simulink model "gm_uz_threephase_VSD_transformation"  (R2021b)
settings: Solver=FixedStepAuto  StartTime=0.0  StopTime=inf  RelTol=1e-3
libraries: hdlmdlgenlib x19, dspsigops x5
settings Model: Creator=ts  LastModifiedBy=valen
settings SolverCC: AlgebraicLoopSolver=TrustRegion  AutoInsertRateTranBlk=on
settings DataIOCC: LimitDataPoints=on  SaveOutput=off  SaveTime=off
settings OptimizationCC: BlockReduction=off  ConditionallyExecuteInputs=off  DefaultParameterBehavior=Inlined  InheritOutputTypeSmallerThanSingle=on  LifeSpan=inf
settings DebuggingCC: AlgebraicLoopMsg=error  InheritedTsInSrcMsg=none  SingleTaskRateTransMsg=error  AllowSymbolicDim=off  StrictBusMsg=ErrorOnBusTreatedAsVector  SFUnexpectedBacktrackingDiag=warning  SFNoUnconditionalDefaultTransitionDiag=warning  SFExecutionAtInitializationDiag=none  SFMachineParentedDataDiag=warning  ArithmeticOperatorsInVariantConditions=warning
settings HardwareCC: ProdBitPerPointer=32  ProdBitPerSizeT=32  ProdBitPerPtrDiffT=32  ProdLargestAtomicFloat=None  ProdIntDivRoundTo=Undefined  ProdEndianess=Unspecified  ProdWordSize=32  ProdHWDeviceType=ASIC/FPGA->ASIC/FPGA  ProdEqTarget=off
settings SFSimCC: SimUseLocalCustomCode=off  CustomCodeUndefinedFunction=UseInterfaceOnly
settings RTWCC: RTWUseLocalCustomCode=off
settings CodeAppCC: StateflowObjectComments=on
settings GRTTargetCC: TargetLangStandard=C89/C90 (ANSI)
settings ConfigComp: CovScope=ReferencedModels  CovMetricSettings=dw  CovSaveCumulativeToWorkspaceVar=on  CovSaveSingleToWorkspaceVar=on  CovExternalEMLEnable=off  CovSFcnEnable=off

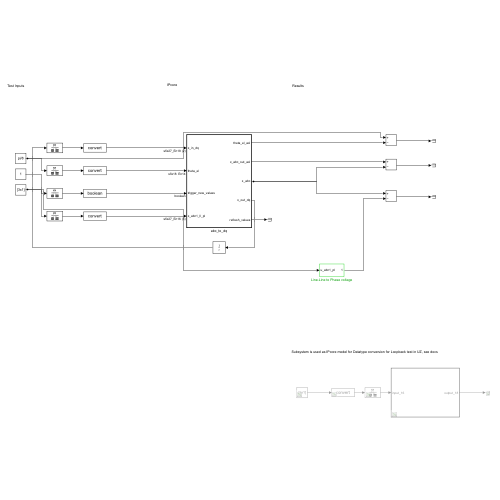
[thumbnail: Simulink's stored preview of the top-level diagram]
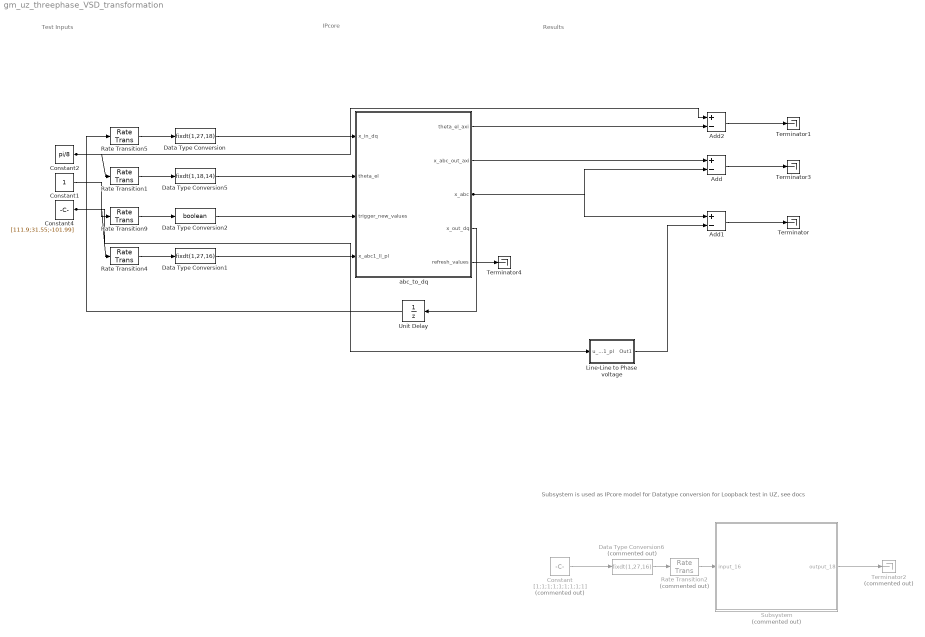
== system gm_uz_threephase_VSD_transformation ==
  note: IPcore
  note: Test Inputs
  note: Results
  note: Subsystem is used as IPcore model for Datatype conversion for Loopback test in UZ, see docs
  Add : Sum  Inputs=+-
  Add1 : Sum  Inputs=+-
  Add2 : Sum  Inputs=+-
  Constant : Constant  Commented=on  Value=[1;1;1;1;1;1;1;1;1]
  Constant1 : Constant
  Constant2 : Constant  Value=pi/8
  Constant4 : Constant  Value=[111.9;31.55;-101.99]
  Data Type Conversion : DataTypeConversion  OutDataTypeStr=fixdt(1,27,18)
  Data Type Conversion1 : DataTypeConversion  OutDataTypeStr=fixdt(1,27,16)
  Data Type Conversion2 : DataTypeConversion  OutDataTypeStr=boolean
  Data Type Conversion5 : DataTypeConversion  OutDataTypeStr=fixdt(1,18,14)
  Data Type Conversion6 : DataTypeConversion  Commented=on  OutDataTypeStr=fixdt(1,27,16)
  Line-Line to Phase voltage : Subsystem
  Rate Transition{1,4..5,9} (4 alike) : RateTransition  OutPortSampleTime=ts_uz_ninephase_VSD_transformation
  Rate Transition2 : RateTransition  Commented=on  OutPortSampleTime=ts_uz_ninephase_VSD_transformation
  Subsystem : Subsystem  Commented=on  TreatAsAtomicUnit=on
  Terminator{,1,3..4} (4 alike) : Terminator
  Terminator2 : Terminator  Commented=on
  Unit Delay : UnitDelay  SampleTime=-1  HasFrameUpgradeWarning=on
  abc_to_dq : Subsystem  TreatAsAtomicUnit=on
  wires:
  abc_to_dq/5(refresh_values) -> Terminator4/1
  Rate Transition2/1 -> Subsystem/1(input_16)
  Data Type Conversion6/1 -> Rate Transition2/1
  Constant/1 -> Data Type Conversion6/1
  Subsystem/1(output_18) -> Terminator2/1
  Line-Line to Phase voltage/1(Out1) -> Add1/2
  Unit Delay/1 -> Rate Transition5/1
  Add/1 -> Terminator3/1
  Constant4/1 -> Rate Transition4/1, Line-Line to Phase voltage/1(u_abc1_pl)
  Add2/1 -> Terminator1/1
  abc_to_dq/1(theta_el_axi) -> Add2/2
  Add1/1 -> Terminator/1
  abc_to_dq/2(x_abc_out_axi) -> Add/1
  abc_to_dq/3(x_abc) -> Add/2, Add1/1
  Constant2/1 -> Rate Transition1/1, Add2/1
  abc_to_dq/4(x_out_dq) -> Unit Delay/1
  Rate Transition1/1 -> Data Type Conversion5/1
  Data Type Conversion5/1 -> abc_to_dq/2(theta_el)
  Constant1/1 -> Rate Transition9/1
  Rate Transition9/1 -> Data Type Conversion2/1
  Data Type Conversion2/1 -> abc_to_dq/3(trigger_new_values)
  Rate Transition4/1 -> Data Type Conversion1/1
  Rate Transition5/1 -> Data Type Conversion/1
  Data Type Conversion1/1 -> abc_to_dq/4(x_abc1_ll_pl)
  Data Type Conversion/1 -> abc_to_dq/1(x_in_dq)

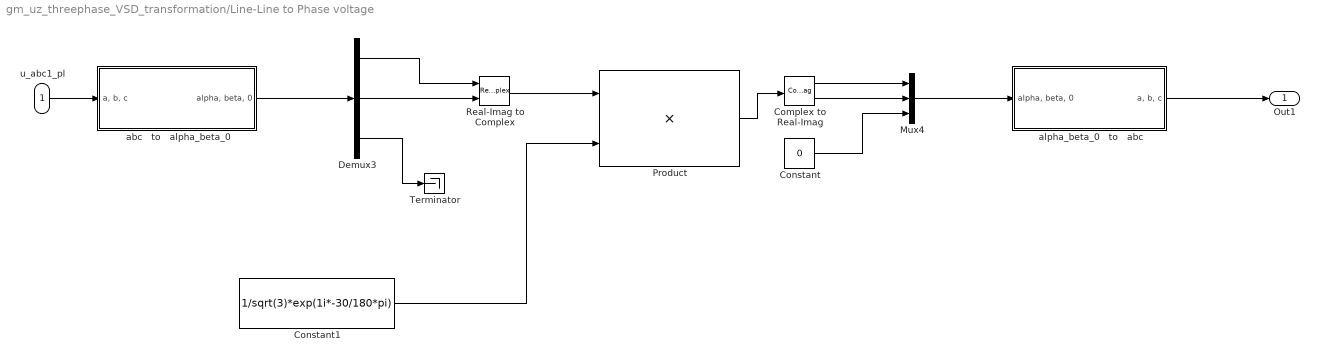
== system gm_uz_threephase_VSD_transformation/Line-Line to Phase voltage ==
  u_abc1_pl : Inport
  Complex to Real-Imag : ComplexToRealImag
  Constant : Constant  Value=0  OutDataTypeStr=fixdt(1,27,16)  SampleTime=-1
  Constant1 : Constant  Value=1/sqrt(3)*exp(1i*-30/180*pi)  OutDataTypeStr=fixdt(1,18,16)  SampleTime=-1
  Demux3 : Demux  Outputs=3
  Mux4 : Mux  Inputs=3
  Product : Product  OutDataTypeStr=fixdt(1,27,16)
  Real-Imag to Complex : RealImagToComplex
  Terminator : Terminator
  abc   to   alpha_beta_0 : Subsystem
  alpha_beta_0   to   abc : Subsystem
  Out1 : Outport
  wires:
  Constant1/1 -> Product/2
  alpha_beta_0   to   abc/1("a, b, c") -> Out1/1
  abc   to   alpha_beta_0/1("alpha, beta, 0 ") -> Demux3/1
  Demux3/3 -> Terminator/1
  u_abc1_pl/1 -> abc   to   alpha_beta_0/1("a, b, c")
  Constant/1 -> Mux4/3
  Complex to Real-Imag/2 -> Mux4/2
  Demux3/1 -> Real-Imag to Complex/1
  Real-Imag to Complex/1 -> Product/1
  Product/1 -> Complex to Real-Imag/1
  Mux4/1 -> alpha_beta_0   to   abc/1("alpha, beta, 0  ")
  Complex to Real-Imag/1 -> Mux4/1
  Demux3/2 -> Real-Imag to Complex/2

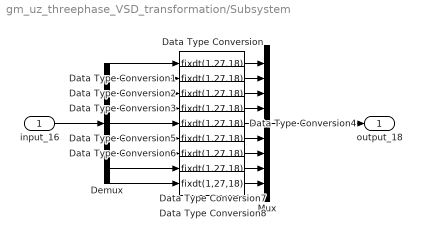
== system gm_uz_threephase_VSD_transformation/Subsystem ==
  input_16 : Inport
  Data Type Conversion{,1..8} (9 alike) : DataTypeConversion  OutDataTypeStr=fixdt(1,27,18)
  Demux : Demux  Outputs=9
  Mux : Mux  Inputs=9
  output_18 : Outport
  wires:
  Mux/1 -> output_18/1
  Data Type Conversion8/1 -> Mux/9
  Data Type Conversion7/1 -> Mux/8
  Data Type Conversion6/1 -> Mux/7
  Data Type Conversion5/1 -> Mux/6
  Data Type Conversion4/1 -> Mux/5
  Data Type Conversion3/1 -> Mux/4
  Data Type Conversion2/1 -> Mux/3
  Data Type Conversion1/1 -> Mux/2
  Data Type Conversion/1 -> Mux/1
  Demux/9 -> Data Type Conversion8/1
  Demux/8 -> Data Type Conversion7/1
  Demux/7 -> Data Type Conversion6/1
  Demux/4 -> Data Type Conversion3/1
  Demux/5 -> Data Type Conversion4/1
  Demux/6 -> Data Type Conversion5/1
  Demux/3 -> Data Type Conversion2/1
  Demux/2 -> Data Type Conversion1/1
  Demux/1 -> Data Type Conversion/1
  input_16/1 -> Demux/1

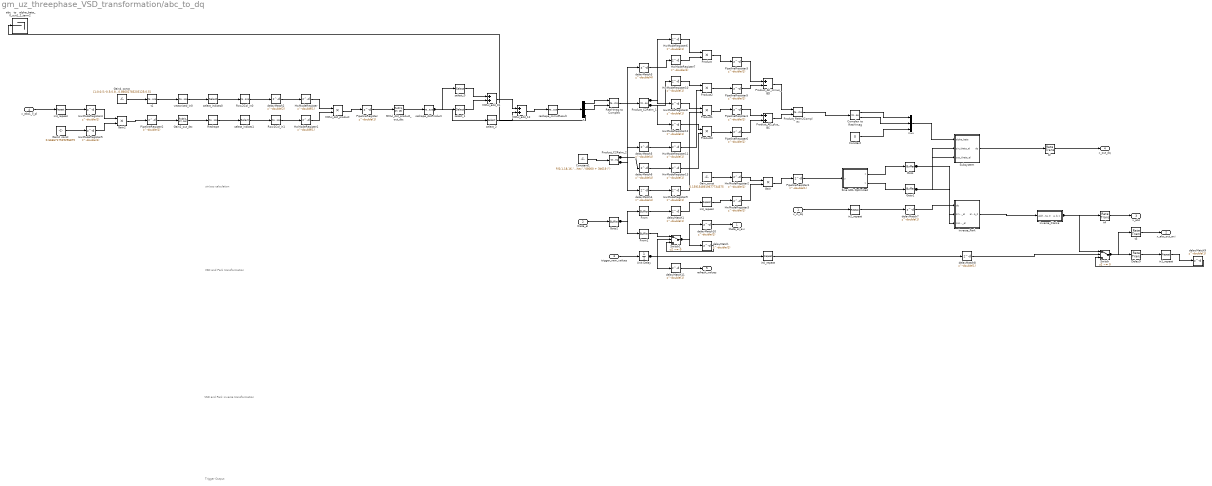
== system gm_uz_threephase_VSD_transformation/abc_to_dq ==
  note: sin/cos calculation
  note: VSD and Park transformation
  note: VSD and Park inverse transformation
  note: Trigger Output
  x_in_dq : Inport  OutDataTypeStr=fixdt(1, 27, 18)  PortDimensions=[2]  SampleTime=1e-06
  theta_el : Inport  Port=2  OutDataTypeStr=fixdt(1, 18, 14)  PortDimensions=1  SampleTime=1e-06
  trigger_new_values : Inport  Port=3  OutDataTypeStr=boolean  PortDimensions=1  SampleTime=1e-06
  x_abc1_ll_pl : Inport  Port=4  OutDataTypeStr=fixdt(1, 27, 16)  PortDimensions=[3]  SampleTime=1e-06
  Complex to Real-Imag : ComplexToRealImag  SampleTime=1e-08
  Constant : Constant  Value=0  OutDataTypeStr=fixdt(1, 27, 16)  SampleTime=1e-08
  Constant1 : Constant  Value="fi(0,1,18,16,\"hex\",\"08000 + 3b619 i\")"  OutDataTypeStr=fixdt(1, 18, 16)  SampleTime=1e-08
  Delay9 : RateTransition  OutPortSampleTimeOpt=Multiple of input port sample time  OutPortSampleTimeMultiple=100
  From : hdlmdlgenlib/Buffer
      settings: SourceProductBaseCode=SL
  From1 : hdlmdlgenlib/Buffer
      settings: SourceProductBaseCode=SL
  Gain : Product  Inputs=**  OutDataTypeStr=fixdt(1, 18, 16)  SampleTime=1e-08
  Gain2 : Product  Inputs=**  OutDataTypeStr=fixdt(1, 45, 32)  SampleTime=1e-08
  Gain2_const : Constant  Value=0.6666717529296875  OutDataTypeStr=fixdt(1, 18, 16)  SampleTime=1e-08
  Gain2_out_dtc : DataTypeConversion  OutDataTypeStr=fixdt(1, 27, 16)  SampleTime=1e-08  SaturateOnIntegerOverflow=on
  Gain4_const : Constant  Value=[1;0;0.5;-0.5;0.86602783203125;0.5;-0.5;-0.86602783203125;0.5]  OutDataTypeStr=fixdt(1, 18, 16)  SampleTime=1e-08
  Gain_const : Constant  Value=0.1591548919677734375  OutDataTypeStr=fixdt(1, 18, 19)  SampleTime=1e-08
  Goto : hdlmdlgenlib/Buffer
      settings: SourceProductBaseCode=SL
  Goto1 : hdlmdlgenlib/Buffer
      settings: SourceProductBaseCode=SL
  Goto2 : hdlmdlgenlib/Buffer
      settings: SourceProductBaseCode=SL
  HwModeRegister{,1..13} (14 alike) : Delay  DelayLength=double(1)  InitialCondition=0  SampleTime=1e-08
  MMul_add_01 : Sum  OutDataTypeStr=fixdt(1, 27, 16)  SaturateOnIntegerOverflow=on  SampleTime=1e-08
  MMul_add_12 : Sum  OutDataTypeStr=fixdt(1, 27, 16)  SaturateOnIntegerOverflow=on  SampleTime=1e-08
  MMul_dot_product : Product  Inputs=**  OutDataTypeStr=fixdt(1, 45, 32)  SampleTime=1e-08
  MMul_dot_product_out_dtc : DataTypeConversion  OutDataTypeStr=fixdt(1, 27, 16)  SampleTime=1e-08  SaturateOnIntegerOverflow=on
  PipelineRegister{,1..6} (7 alike) : Delay  DelayLength=double(1)  InitialCondition=0  SampleTime=1e-08
  Product{,1..3} (4 alike) : Product  Inputs=**  OutDataTypeStr=fixdt(1, 27, 16)  SampleTime=1e-08
  Product_AC_minus_BD : Sum  Inputs=+-  OutDataTypeStr=fixdt(1, 27, 16)  SampleTime=1e-08
  Product_AD_plus_BC : Sum  OutDataTypeStr=fixdt(1, 27, 16)  SampleTime=1e-08
  Product_C2ReIm_1 : ComplexToRealImag  SampleTime=1e-08
  Product_C2ReIm_2 : ComplexToRealImag  SampleTime=1e-08
  Product_ReIm2Complex : RealImagToComplex  SampleTime=1e-08
  Real-Imag to Complex : RealImagToComplex  ConstantPart="fi(0,1,27,16,\"hex\",\"0000000\")"  SampleTime=1e-08
  Reshape : Reshape  OutputDimensionality=Column vector (2-D)
  Row2Col_in0 : Reshape  OutputDimensionality=Column vector (2-D)
  Row2Col_in1 : Reshape  OutputDimensionality=Column vector (2-D)
  Sine HDL Optimized : Subsystem  mask(Sine and Cosine HDL optimized block){OutputFormula=sin(2*pi*u) and cos(2*pi*u), NumDataPoints=double(256), TableDataTypeStr=fixdt(0,17,16), SimulateLUTROMDelay=off}
      mask prompts: OutputFormula "Simulink:masks:OutputFormula_MP"; NumDataPoints "HDLShared:hdlshared:CosineHDL_Npts"; TableDataTypeStr "Simulink:blkprm_prompts:TABLE_UNIFIEDDATATYPE"; SimulateLUTROMDelay "HDLShared:hdlshared:CosineHDL_SimulateLUTDelay"
      mask help: Sine and Cosine HDL optimized block using quarter wave symmetry, and HDL friendly settings.
      mask Help: helpview([docroot '/hdlcoder/helptargets.map'],'SineAndCosineHDL_Optimized');
      mask TypeOptions OutputFormula: sin(2*pi*u) | cos(2*pi*u) | exp(j*2*pi*u) | sin(2*pi*u) and cos(2*pi*u)
      mask Display:
      | port_label('input',1,'u')
      | port_label('output',1,'sin(2*pi*u)')
      | port_label('output',2,'cos(2*pi*u)')
      | xpos = 0.35;
      | yoffset = 0.5;
      | if ( SimulateLUTROMDelay )
      |   text(xpos,yoffset,'HDL (Z^{-1})','texmode','on')
      | else
      |    text(xpos,yoffset,'HDL')
      | end
  Subsystem : Subsystem
  Switch : Switch  Criteria=u2 ~= 0  Threshold=double(0)  OutDataTypeStr=fixdt(1, 27, 18)  SampleTime=1e-08
  Switch1 : Switch  Criteria=u2 ~= 0  Threshold=double(0)  OutDataTypeStr=fixdt(1, 18, 14)  SampleTime=1e-06
  Unit Delay : UnitDelay  SampleTime=1e-06
  abc   to   alpha_beta_0_out1_2_term2 : Terminator
  delayMatch{,1,10..11} (4 alike) : Delay  DelayLength=double(1)  InitialCondition=0  SampleTime=1e-06
  delayMatch2 : Delay  DelayLength=double(2)  InitialCondition=0  SampleTime=1e-08
  delayMatch{3..6} (4 alike) : Delay  DelayLength=double(4)  InitialCondition=0  SampleTime=1e-08
  delayMatch7 : Delay  DelayLength=double(1)  InitialCondition=0  SampleTime=1e-08
  delayMatch8 : Delay  DelayLength=double(1)  InitialCondition=0  SampleTime=1e-08
  delayMatch9 : Delay  DelayLength=double(1)  InitialCondition=0  SampleTime=1e-08
  in0_repeat : dspsigops/Repeat  N=double(100)  RateOptions=Allow multirate processing  ic=0  mode=Unused parameter value
  in1_repeat : dspsigops/Repeat  N=double(100)  RateOptions=Allow multirate processing  ic=0  mode=Unused parameter value
  in2_repeat : dspsigops/Repeat  N=double(100)  RateOptions=Allow multirate processing  ic=0  mode=Unused parameter value
  in3_repeat : dspsigops/Repeat  N=double(100)  RateOptions=Allow multirate processing  ic=0  mode=Unused parameter value
  in4_repeat : dspsigops/Repeat  N=double(100)  RateOptions=Allow multirate processing  ic=0  mode=Unused parameter value
  inverse_Clarke : Subsystem
  inverse_Park : Subsystem
  mux : Mux  Inputs=3
  reshape_dotProduct : Reshape  OutputDimensionality=Customize  OutputDimensions=[3,3]
  reshape_mmulResult : Reshape  OutputDimensionality=Customize  OutputDimensions=[3,1]
  select_0 : Selector  NumberOfDimensions=2  SampleTime=1e-08  IndexOptions=Index vector (dialog),Select all  Indices=double(1),[]  OutputSizes=1
  select_1 : Selector  NumberOfDimensions=2  SampleTime=1e-08  IndexOptions=Index vector (dialog),Select all  Indices=double(2),[]  OutputSizes=1
  select_2 : Selector  NumberOfDimensions=2  SampleTime=1e-08  IndexOptions=Index vector (dialog),Select all  Indices=double(3),[]  OutputSizes=1
  select_indices0 : Selector  SampleTime=1e-08  IndexOptions=Index vector (dialog)  Indices=double([1 4 7 2 5 8 3 6 9])  OutputSizes=1
  select_indices1 : Selector  SampleTime=1e-08  IndexOptions=Index vector (dialog)  Indices=double([1 2 3 1 2 3 1 2 3])  OutputSizes=1
  t : Demux  Outputs=3
  t1 : Reshape  OutputDimensionality=Customize  OutputDimensions=[3,3]
  t2 : RateTransition  OutPortSampleTimeOpt=Multiple of input port sample time  OutPortSampleTimeMultiple=100
  t3 : RateTransition  OutPortSampleTimeOpt=Multiple of input port sample time  OutPortSampleTimeMultiple=100
  t4 : RateTransition  OutPortSampleTimeOpt=Multiple of input port sample time  OutPortSampleTimeMultiple=100
  vectorized_in0 : Reshape  OutputDimensionality=Row vector (2-D)
  theta_el_axi : Outport  SampleTime=1e-06
  x_abc_out_axi : Outport  Port=2  SampleTime=1e-06
  x_abc : Outport  Port=3  SampleTime=1e-06
  x_out_dq : Outport  Port=4  SampleTime=1e-06
  refresh_values : Outport  Port=5  SampleTime=1e-06
  wires:
  x_in_dq/1 -> in2_repeat/1
  theta_el/1 -> Goto2/1
  trigger_new_values/1 -> Unit Delay/1
  x_abc1_ll_pl/1 -> in4_repeat/1
  delayMatch1/1 -> in3_repeat/1
  delayMatch11/1 -> refresh_values/1
  delayMatch10/1 -> theta_el_axi/1
  t2/1 -> x_out_dq/1
  t3/1 -> x_abc_out_axi/1
  t4/1 -> x_abc/1
  Switch1/1 -> delayMatch10/1, delayMatch/1
  Unit Delay/1 -> delayMatch11/1, Switch1/2, in0_repeat/1
  delayMatch/1 -> Switch1/3
  Delay9/1 -> in1_repeat/1
  Goto2/1 -> From1/1, From/1
  From1/1 -> Switch1/1
  From/1 -> delayMatch1/1
  Subsystem/1(dq) -> t2/1
  Switch/1 -> t3/1, Delay9/1
  inverse_Clarke/1("a, b, c") -> t4/1, Switch/1
  in0_repeat/1 -> delayMatch8/1
  in1_repeat/1 -> delayMatch9/1
  in2_repeat/1 -> delayMatch7/1
  in3_repeat/1 -> HwModeRegister3/1
  in4_repeat/1 -> HwModeRegister4/1
  PipelineRegister1/1 -> Sine HDL Optimized/1(u)
  Sine HDL Optimized/1(x) -> Goto/1
  Sine HDL Optimized/2(y) -> Goto1/1
  inverse_Park/1(alpha_beta_0) -> inverse_Clarke/1("alpha, beta, 0  ")
  Constant/1 -> mux/3
  mux/1 -> Subsystem/1(alpha_beta)
  Gain2_out_dtc/1 -> Reshape/1
  Reshape/1 -> select_indices1/1
  reshape_mmulResult/1 -> t/1
  Real-Imag to Complex/1 -> Product_C2ReIm_1/1
  Constant1/1 -> Product_C2ReIm_2/1
  Product_ReIm2Complex/1 -> Complex to Real-Imag/1
  Complex to Real-Imag/1 -> mux/1
  Complex to Real-Imag/2 -> mux/2
  delayMatch8/1 -> Switch/2
  delayMatch9/1 -> Switch/3
  delayMatch7/1 -> inverse_Park/1(dq)
  t/1 -> Real-Imag to Complex/1
  t/2 -> Real-Imag to Complex/2
  t/3 -> abc   to   alpha_beta_0_out1_2_term2/1
  t1/1 -> vectorized_in0/1
  vectorized_in0/1 -> select_indices0/1
  select_indices0/1 -> Row2Col_in0/1
  select_indices1/1 -> Row2Col_in1/1
  delayMatch2/1 -> HwModeRegister/1
  Row2Col_in1/1 -> HwModeRegister1/1
  MMul_dot_product_out_dtc/1 -> reshape_dotProduct/1
  reshape_dotProduct/1 -> select_2/1, select_1/1, select_0/1
  select_0/1 -> MMul_add_01/1
  select_1/1 -> MMul_add_01/2
  MMul_add_01/1 -> MMul_add_12/1
  select_2/1 -> MMul_add_12/2
  MMul_add_12/1 -> reshape_mmulResult/1
  Gain4_const/1 -> t1/1
  Gain_const/1 -> HwModeRegister2/1
  Gain2_const/1 -> HwModeRegister5/1
  Product_C2ReIm_1/1 -> HwModeRegister6/1, HwModeRegister8/1
  Product_C2ReIm_1/2 -> HwModeRegister10/1, HwModeRegister12/1
  delayMatch3/1 -> HwModeRegister7/1
  delayMatch4/1 -> HwModeRegister9/1
  PipelineRegister3/1 -> Product_AC_minus_BD/1
  PipelineRegister4/1 -> Product_AD_plus_BC/1
  PipelineRegister5/1 -> Product_AC_minus_BD/2
  PipelineRegister6/1 -> Product_AD_plus_BC/2
  Product_AC_minus_BD/1 -> Product_ReIm2Complex/1
  Product_AD_plus_BC/1 -> Product_ReIm2Complex/2
  PipelineRegister/1 -> MMul_dot_product_out_dtc/1
  PipelineRegister2/1 -> Gain2_out_dtc/1
  Row2Col_in0/1 -> delayMatch2/1
  delayMatch6/1 -> HwModeRegister13/1
  delayMatch5/1 -> HwModeRegister11/1
  Product_C2ReIm_2/2 -> delayMatch5/1, delayMatch4/1
  Product_C2ReIm_2/1 -> delayMatch6/1, delayMatch3/1
  Goto/1 -> inverse_Park/2(sin_theta_el), Subsystem/2(sin_theta_el)
  Goto1/1 -> inverse_Park/3(cos_theta_el), Subsystem/3(cos_theta_el)
  MMul_dot_product/1 -> PipelineRegister/1
  HwModeRegister/1 -> MMul_dot_product/1
  HwModeRegister1/1 -> MMul_dot_product/2
  Gain/1 -> PipelineRegister1/1
  HwModeRegister2/1 -> Gain/1
  HwModeRegister3/1 -> Gain/2
  Gain2/1 -> PipelineRegister2/1
  HwModeRegister4/1 -> Gain2/1
  HwModeRegister5/1 -> Gain2/2
  Product/1 -> PipelineRegister3/1
  HwModeRegister6/1 -> Product/1
  HwModeRegister7/1 -> Product/2
  Product1/1 -> PipelineRegister4/1
  HwModeRegister8/1 -> Product1/1
  HwModeRegister9/1 -> Product1/2
  Product2/1 -> PipelineRegister5/1
  HwModeRegister10/1 -> Product2/1
  HwModeRegister11/1 -> Product2/2
  Product3/1 -> PipelineRegister6/1
  HwModeRegister12/1 -> Product3/1
  HwModeRegister13/1 -> Product3/2

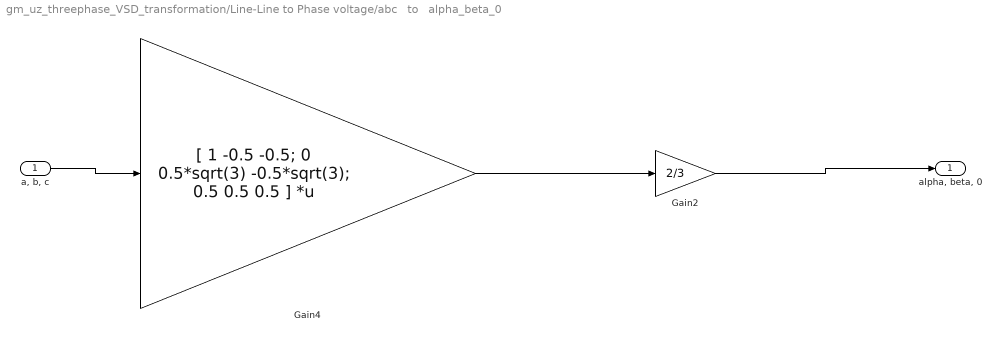
== system gm_uz_threephase_VSD_transformation/Line-Line to Phase voltage/abc   to   alpha_beta_0 ==
  "a, b, c" : Inport  PortDimensions=3
  Gain2 : Gain  Gain=2/3  ParamDataTypeStr=fixdt(1,18,16)  SaturateOnIntegerOverflow=on  OutDataTypeStr=Inherit: Same as input
  Gain4 : Gain  Gain="[ 1   -0.5   -0.5; 0   0.5*sqrt(3)   -0.5*sqrt(3); 0.5  0.5  0.5 ]"  Multiplication=Matrix(K*u) (u vector)  ParamDataTypeStr=fixdt(1,18,16)  OutDataTypeStr=fixdt(1,27,16)  SaturateOnIntegerOverflow=on
  "alpha, beta, 0 " : Outport
  wires:
  Gain4/1 -> Gain2/1
  "a, b, c"/1 -> Gain4/1
  Gain2/1 -> "alpha, beta, 0 "/1

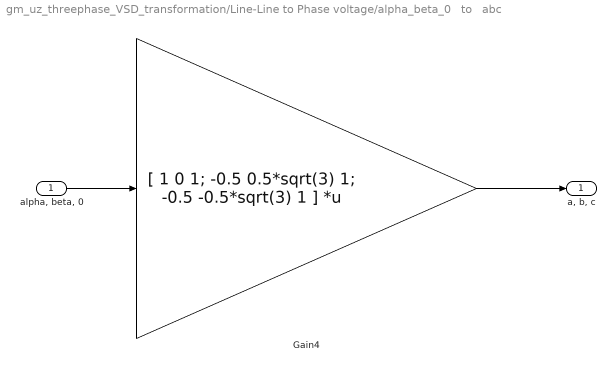
== system gm_uz_threephase_VSD_transformation/Line-Line to Phase voltage/alpha_beta_0   to   abc ==
  "alpha, beta, 0  " : Inport  PortDimensions=3
  Gain4 : Gain  Gain="[ 1 0 1; -0.5   0.5*sqrt(3)  1; -0.5 -0.5*sqrt(3) 1 ]"  Multiplication=Matrix(K*u) (u vector)  ParamDataTypeStr=fixdt(1,18,16)  SaturateOnIntegerOverflow=on  OutDataTypeStr=Inherit: Same as input
  "a, b, c" : Outport
  wires:
  "alpha, beta, 0  "/1 -> Gain4/1
  Gain4/1 -> "a, b, c"/1

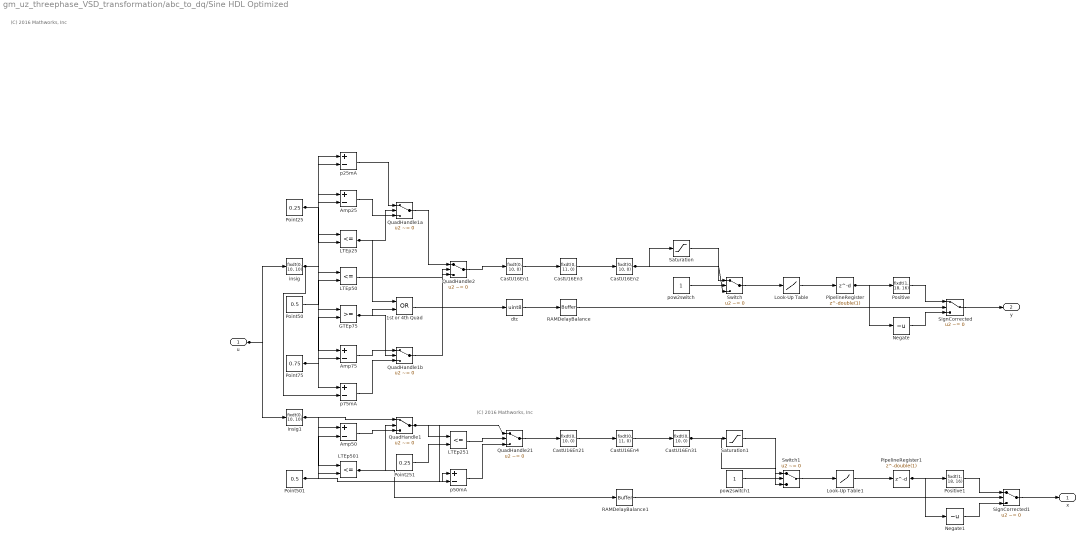
== system gm_uz_threephase_VSD_transformation/abc_to_dq/Sine HDL Optimized ==
  note: (C) 2016 Mathworks, Inc
  note: (C) 2016 Mathworks, Inc
  u : Inport  OutDataTypeStr=fixdt(1, 18, 16)  SampleTime=1e-08
  1st or 4th Quad : Logic  Operator=OR  AllPortsSameDT=off  OutDataTypeStr=boolean  SampleTime=1e-08
  Amp25 : Sum  Inputs=+-  AccumDataTypeStr=fixdt(1, 19, 18)  OutDataTypeStr=fixdt(1, 19, 18)  SampleTime=1e-08
  Amp50 : Sum  Inputs=+-  AccumDataTypeStr=fixdt(1, 19, 18)  OutDataTypeStr=fixdt(1, 19, 18)  SampleTime=1e-08
  Amp75 : Sum  Inputs=+-  AccumDataTypeStr=fixdt(1, 19, 18)  OutDataTypeStr=fixdt(1, 19, 18)  SampleTime=1e-08
  CastU16En1 : DataTypeConversion  OutDataTypeStr=fixdt(0, 10, 0)  ConvertRealWorld=Stored Integer (SI)  SampleTime=1e-08
  CastU16En2 : DataTypeConversion  OutDataTypeStr=fixdt(0, 10, 0)  ConvertRealWorld=Stored Integer (SI)  SampleTime=1e-08  SaturateOnIntegerOverflow=on
  CastU16En21 : DataTypeConversion  OutDataTypeStr=fixdt(0, 10, 0)  ConvertRealWorld=Stored Integer (SI)  SampleTime=1e-08
  CastU16En3 : DataTypeConversion  OutDataTypeStr=fixdt(0, 11, 0)  SampleTime=1e-08
  CastU16En31 : DataTypeConversion  OutDataTypeStr=fixdt(0, 10, 0)  ConvertRealWorld=Stored Integer (SI)  SampleTime=1e-08  SaturateOnIntegerOverflow=on
  CastU16En4 : DataTypeConversion  OutDataTypeStr=fixdt(0, 11, 0)  SampleTime=1e-08
  GTEp75 : RelationalOperator  OutDataTypeStr=boolean  SampleTime=1e-08  RndMeth=Nearest
  LTEp{25,50,251,501} (4 alike) : RelationalOperator  Operator=<=  OutDataTypeStr=boolean  SampleTime=1e-08  RndMeth=Nearest
  Look-Up Table : Lookup_n-D  NumberOfTableDimensions=1  BreakpointsForDimension1="fi(\"numerictype\",numerictype(0,10,0),\"fimath\",fimath(\"RoundingMethod\", \"Floor\",\"OverflowAction\", \"Wrap\",\"ProductMode\",\"FullPrecision\",\"SumMode\",\"FullPrecision\"),\"Value\",\"[0 1 2 3 4 5 6 7 8 9 10 11 12 13 14 15 16 17 18 19 20 21 22 23 24 25 26 27 28 29 30 31 32 33 34 35 36 37 38 39 40 41 42 43 44 45 46 47 48 49 50 51 52 53 54 55 56 57 58 59 60 61 62 63 64 65 66 67 68 69 70 71 72 73 74 75 76 77 78 79 80 81 82 83 84 85 86 87 88 89 90 91 92 93 94 95 96 97 98 99 100 101 102 103 104 105 106 107 108 109 110 111 112 113 114 115 116 117 118 119 120 121 122 123 124 125 126 127 128 129 130 131 132 133 134 135 136 137 138 139 140 141 142 143 144 145 146 147 148 149 150 151 152 153 154 155 156 157 158 159 160 161 162 163 164 165 166 167 168 169 170 171 172 173 174 175 176 177 178 179 180 181 182 183 184 185 186 187 188 189 190 191 192 193 194 195 196 197 198 199 200 201 202 203 204 205 206 207 208 209 210 211 212 213 214 215 216 217 218 219 220 221 222 223 224 225 226 227 228 229 230 231 232 233 234 235 236 237 238 239 240 241 242 243 244 245 246 247 248 249 250 251 252 253 254 255]\")"  Table="reshape(fi(\"numerictype\",numerictype(1,18,16),\"fimath\",fimath(\"RoundingMethod\", \"Floor\",\"OverflowAction\", \"Wrap\",\"ProductMode\",\"FullPrecision\",\"SumMode\",\"FullPrecision\"),\"Value\",\"[0;0.006134033203125;0.01226806640625;0.018402099609375;0.0245361328125;0.030670166015625;0.03680419921875;0.042938232421875;0.049072265625;0.0551910400390625;0.0613250732421875;0.06744384765625;0.0735626220703125;0.079681396484375;0.0858001708984375;0.0919036865234375;0.0980224609375;0.1041259765625;0.1102294921875;0.1163177490234375;0.122406005859375;0.1284942626953125;0.13458251953125;0.140655517578125;0.146728515625;0.152801513671875;0.1588592529296875;0.1649169921875;0.17095947265625;0.177001953125;0.18304443359375;0.1890716552734375;0.1950836181640625;0.20111083984375;0.2071075439453125;0.213104248046875;0.2191009521484375;0.2250823974609375;0.2310638427734375;0.237030029296875;0.24298095703125;0.248931884765625;0.2548675537109375;0.2607879638671875;0.2667083740234375;0.2726287841796875;0.2785186767578125;0.2844085693359375;0.290283203125;0.2961578369140625;0.302001953125;0.3078460693359375;0.3136749267578125;0.3195037841796875;0.3253173828125;0.3311004638671875;0.336883544921875;0.3426666259765625;0.348419189453125;0.354156494140625;0.359893798828125;0.3656158447265625;0.3713226318359375;0.37701416015625;0.3826904296875;0.3883514404296875;0.3939971923828125;0.399627685546875;0.405242919921875;0.4108428955078125;0.4164276123046875;0.4219970703125;0.42755126953125;0.4330902099609375;0.4386138916015625;0.444122314453125;0.449615478515625;0.455078125;0.460540771484375;0.465972900390625;0.4713897705078125;0.476806640625;0.482177734375;0.487548828125;0.4929046630859375;0.49822998046875;0.5035400390625;0.5088348388671875;0.51409912109375;0.5193634033203125;0.52459716796875;0.5298004150390625;0.535003662109375;0.5401763916015625;0.545318603515625;0.5504608154296875;0.555572509765625;0.5606689453125;0.56573486328125;0.5707855224609375;0.5758056640625;0.580810546875;0.5858001708984375;0.59075927734375;0.595703125;0.600616455078125;0.6055145263671875;0.610382080078125;0.615234375;0.62005615234375;0.6248626708984375;0.629638671875;0.6343994140625;0.639129638671875;0.643829345703125;0.6485137939453125;0.653167724609375;0.657806396484375;0.66241455078125;0.6670074462890625;0.6715545654296875;0.67608642578125;0.68060302734375;0.685089111328125;0.689544677734375;0.6939697265625;0.6983795166015625;0.7027587890625;0.7071075439453125;0.71142578125;0.715728759765625;0.720001220703125;0.7242431640625;0.7284698486328125;0.7326507568359375;0.73681640625;0.7409515380859375;0.74505615234375;0.7491302490234375;0.7531890869140625;0.7572021484375;0.761199951171875;0.765167236328125;0.76910400390625;0.77301025390625;0.776885986328125;0.780731201171875;0.7845611572265625;0.7883453369140625;0.7920989990234375;0.79583740234375;0.799530029296875;0.8032073974609375;0.806854248046875;0.810455322265625;0.8140411376953125;0.8175811767578125;0.82110595703125;0.8245849609375;0.8280487060546875;0.8314666748046875;0.834869384765625;0.838226318359375;0.841552734375;0.8448486328125;0.848114013671875;0.851348876953125;0.85455322265625;0.85772705078125;0.860870361328125;0.8639678955078125;0.8670501708984375;0.870086669921875;0.8730926513671875;0.876068115234375;0.8790130615234375;0.881927490234375;0.884796142578125;0.88763427734375;0.89044189453125;0.893218994140625;0.895965576171875;0.898681640625;0.9013519287109375;0.90399169921875;0.9066009521484375;0.9091644287109375;0.911712646484375;0.914215087890625;0.9166717529296875;0.9191131591796875;0.9215087890625;0.9238739013671875;0.92620849609375;0.9285125732421875;0.9307708740234375;0.9329986572265625;0.9351806640625;0.9373321533203125;0.939453125;0.9415435791015625;0.9435882568359375;0.9456024169921875;0.9475860595703125;0.94952392578125;0.9514312744140625;0.95330810546875;0.95513916015625;0.956939697265625;0.958709716796875;0.9604339599609375;0.962127685546875;0.963775634765625;0.96539306640625;0.96697998046875;0.9685211181640625;0.97003173828125;0.97149658203125;0.9729461669921875;0.974334716796875;0.9757080078125;0.9770355224609375;0.9783172607421875;0.9795684814453125;0.9807891845703125;0.981964111328125 ...(+541 chars)]\"), [1  256])"  InterpMethod=Flat  ExtrapMethod=Clip  DiagnosticForOutOfRangeInput=Error  SampleTime=1e-08  OutDataTypeStr=fixdt(1, 18, 16)  InputSameDT=on
  Look-Up Table1 : Lookup_n-D  NumberOfTableDimensions=1  BreakpointsForDimension1="fi(\"numerictype\",numerictype(0,10,0),\"fimath\",fimath(\"RoundingMethod\", \"Floor\",\"OverflowAction\", \"Wrap\",\"ProductMode\",\"FullPrecision\",\"SumMode\",\"FullPrecision\"),\"Value\",\"[0 1 2 3 4 5 6 7 8 9 10 11 12 13 14 15 16 17 18 19 20 21 22 23 24 25 26 27 28 29 30 31 32 33 34 35 36 37 38 39 40 41 42 43 44 45 46 47 48 49 50 51 52 53 54 55 56 57 58 59 60 61 62 63 64 65 66 67 68 69 70 71 72 73 74 75 76 77 78 79 80 81 82 83 84 85 86 87 88 89 90 91 92 93 94 95 96 97 98 99 100 101 102 103 104 105 106 107 108 109 110 111 112 113 114 115 116 117 118 119 120 121 122 123 124 125 126 127 128 129 130 131 132 133 134 135 136 137 138 139 140 141 142 143 144 145 146 147 148 149 150 151 152 153 154 155 156 157 158 159 160 161 162 163 164 165 166 167 168 169 170 171 172 173 174 175 176 177 178 179 180 181 182 183 184 185 186 187 188 189 190 191 192 193 194 195 196 197 198 199 200 201 202 203 204 205 206 207 208 209 210 211 212 213 214 215 216 217 218 219 220 221 222 223 224 225 226 227 228 229 230 231 232 233 234 235 236 237 238 239 240 241 242 243 244 245 246 247 248 249 250 251 252 253 254 255]\")"  Table="reshape(fi(\"numerictype\",numerictype(1,18,16),\"fimath\",fimath(\"RoundingMethod\", \"Floor\",\"OverflowAction\", \"Wrap\",\"ProductMode\",\"FullPrecision\",\"SumMode\",\"FullPrecision\"),\"Value\",\"[0;0.006134033203125;0.01226806640625;0.018402099609375;0.0245361328125;0.030670166015625;0.03680419921875;0.042938232421875;0.049072265625;0.0551910400390625;0.0613250732421875;0.06744384765625;0.0735626220703125;0.079681396484375;0.0858001708984375;0.0919036865234375;0.0980224609375;0.1041259765625;0.1102294921875;0.1163177490234375;0.122406005859375;0.1284942626953125;0.13458251953125;0.140655517578125;0.146728515625;0.152801513671875;0.1588592529296875;0.1649169921875;0.17095947265625;0.177001953125;0.18304443359375;0.1890716552734375;0.1950836181640625;0.20111083984375;0.2071075439453125;0.213104248046875;0.2191009521484375;0.2250823974609375;0.2310638427734375;0.237030029296875;0.24298095703125;0.248931884765625;0.2548675537109375;0.2607879638671875;0.2667083740234375;0.2726287841796875;0.2785186767578125;0.2844085693359375;0.290283203125;0.2961578369140625;0.302001953125;0.3078460693359375;0.3136749267578125;0.3195037841796875;0.3253173828125;0.3311004638671875;0.336883544921875;0.3426666259765625;0.348419189453125;0.354156494140625;0.359893798828125;0.3656158447265625;0.3713226318359375;0.37701416015625;0.3826904296875;0.3883514404296875;0.3939971923828125;0.399627685546875;0.405242919921875;0.4108428955078125;0.4164276123046875;0.4219970703125;0.42755126953125;0.4330902099609375;0.4386138916015625;0.444122314453125;0.449615478515625;0.455078125;0.460540771484375;0.465972900390625;0.4713897705078125;0.476806640625;0.482177734375;0.487548828125;0.4929046630859375;0.49822998046875;0.5035400390625;0.5088348388671875;0.51409912109375;0.5193634033203125;0.52459716796875;0.5298004150390625;0.535003662109375;0.5401763916015625;0.545318603515625;0.5504608154296875;0.555572509765625;0.5606689453125;0.56573486328125;0.5707855224609375;0.5758056640625;0.580810546875;0.5858001708984375;0.59075927734375;0.595703125;0.600616455078125;0.6055145263671875;0.610382080078125;0.615234375;0.62005615234375;0.6248626708984375;0.629638671875;0.6343994140625;0.639129638671875;0.643829345703125;0.6485137939453125;0.653167724609375;0.657806396484375;0.66241455078125;0.6670074462890625;0.6715545654296875;0.67608642578125;0.68060302734375;0.685089111328125;0.689544677734375;0.6939697265625;0.6983795166015625;0.7027587890625;0.7071075439453125;0.71142578125;0.715728759765625;0.720001220703125;0.7242431640625;0.7284698486328125;0.7326507568359375;0.73681640625;0.7409515380859375;0.74505615234375;0.7491302490234375;0.7531890869140625;0.7572021484375;0.761199951171875;0.765167236328125;0.76910400390625;0.77301025390625;0.776885986328125;0.780731201171875;0.7845611572265625;0.7883453369140625;0.7920989990234375;0.79583740234375;0.799530029296875;0.8032073974609375;0.806854248046875;0.810455322265625;0.8140411376953125;0.8175811767578125;0.82110595703125;0.8245849609375;0.8280487060546875;0.8314666748046875;0.834869384765625;0.838226318359375;0.841552734375;0.8448486328125;0.848114013671875;0.851348876953125;0.85455322265625;0.85772705078125;0.860870361328125;0.8639678955078125;0.8670501708984375;0.870086669921875;0.8730926513671875;0.876068115234375;0.8790130615234375;0.881927490234375;0.884796142578125;0.88763427734375;0.89044189453125;0.893218994140625;0.895965576171875;0.898681640625;0.9013519287109375;0.90399169921875;0.9066009521484375;0.9091644287109375;0.911712646484375;0.914215087890625;0.9166717529296875;0.9191131591796875;0.9215087890625;0.9238739013671875;0.92620849609375;0.9285125732421875;0.9307708740234375;0.9329986572265625;0.9351806640625;0.9373321533203125;0.939453125;0.9415435791015625;0.9435882568359375;0.9456024169921875;0.9475860595703125;0.94952392578125;0.9514312744140625;0.95330810546875;0.95513916015625;0.956939697265625;0.958709716796875;0.9604339599609375;0.962127685546875;0.963775634765625;0.96539306640625;0.96697998046875;0.9685211181640625;0.97003173828125;0.97149658203125;0.9729461669921875;0.974334716796875;0.9757080078125;0.9770355224609375;0.9783172607421875;0.9795684814453125;0.9807891845703125;0.981964111328125 ...(+541 chars)]\"), [1  256])"  InterpMethod=Flat  ExtrapMethod=Clip  DiagnosticForOutOfRangeInput=Error  SampleTime=1e-08  OutDataTypeStr=fixdt(1, 18, 16)  InputSameDT=on
  Negate : UnaryMinus  SampleTime=1e-08
  Negate1 : UnaryMinus  SampleTime=1e-08
  PipelineRegister : Delay  DelayLength=double(1)  InitialCondition=0  SampleTime=1e-08
  PipelineRegister1 : Delay  DelayLength=double(1)  InitialCondition=0  SampleTime=1e-08
  Point25 : Constant  Value=0.25  OutDataTypeStr=fixdt(0, 18, 18)  SampleTime=1e-08
  Point251 : Constant  Value=0.25  OutDataTypeStr=fixdt(0, 18, 18)  SampleTime=1e-08
  Point50 : Constant  Value=0.5  OutDataTypeStr=fixdt(0, 18, 18)  SampleTime=1e-08
  Point501 : Constant  Value=0.5  OutDataTypeStr=fixdt(0, 18, 18)  SampleTime=1e-08
  Point75 : Constant  Value=0.75  OutDataTypeStr=fixdt(0, 18, 18)  SampleTime=1e-08
  Positive : DataTypeConversion  OutDataTypeStr=fixdt(1, 18, 16)  SampleTime=1e-08
  Positive1 : DataTypeConversion  OutDataTypeStr=fixdt(1, 18, 16)  SampleTime=1e-08
  QuadHandle1 : Switch  Criteria=u2 ~= 0  Threshold=double(0)  OutDataTypeStr=fixdt(1, 19, 18)  SampleTime=1e-08
  QuadHandle1a : Switch  Criteria=u2 ~= 0  Threshold=double(0)  OutDataTypeStr=fixdt(1, 19, 18)  SampleTime=1e-08
  QuadHandle1b : Switch  Criteria=u2 ~= 0  Threshold=double(0)  OutDataTypeStr=fixdt(1, 19, 18)  SampleTime=1e-08
  QuadHandle2 : Switch  Criteria=u2 ~= 0  Threshold=double(0)  OutDataTypeStr=fixdt(0, 10, 10)  SampleTime=1e-08  SaturateOnIntegerOverflow=on
  QuadHandle21 : Switch  Criteria=u2 ~= 0  Threshold=double(0)  OutDataTypeStr=fixdt(0, 10, 10)  SampleTime=1e-08
  RAMDelayBalance : hdlmdlgenlib/Buffer
      settings: SourceProductBaseCode=SL
  RAMDelayBalance1 : hdlmdlgenlib/Buffer
      settings: SourceProductBaseCode=SL
  Saturation : Saturate  UpperLimit="fi(0,0,10,0,\"hex\",\"0ff\")"  LowerLimit="fi(0,0,10,0,\"hex\",\"000\")"  SampleTime=1e-08  OutDataTypeStr=fixdt(0, 10, 0)
  Saturation1 : Saturate  UpperLimit="fi(0,0,10,0,\"hex\",\"0ff\")"  LowerLimit="fi(0,0,10,0,\"hex\",\"000\")"  SampleTime=1e-08  OutDataTypeStr=fixdt(0, 10, 0)
  SignCorrected : Switch  Criteria=u2 ~= 0  Threshold=double(0)  OutDataTypeStr=fixdt(1, 18, 16)  SampleTime=1e-08
  SignCorrected1 : Switch  Criteria=u2 ~= 0  Threshold=double(0)  OutDataTypeStr=fixdt(1, 18, 16)  SampleTime=1e-08
  Switch : Switch  Criteria=u2 ~= 0  Threshold=double(0)  OutDataTypeStr=fixdt(0, 10, 0)  SampleTime=1e-08
  Switch1 : Switch  Criteria=u2 ~= 0  Threshold=double(0)  OutDataTypeStr=fixdt(0, 10, 0)  SampleTime=1e-08
  dtc : DataTypeConversion  OutDataTypeStr=uint8  SampleTime=1e-08
  insig : DataTypeConversion  OutDataTypeStr=fixdt(0, 10, 10)  SampleTime=1e-08
  insig1 : DataTypeConversion  OutDataTypeStr=fixdt(0, 10, 10)  SampleTime=1e-08
  p25mA : Sum  Inputs=+-  AccumDataTypeStr=fixdt(1, 19, 18)  OutDataTypeStr=fixdt(1, 19, 18)  SampleTime=1e-08
  p50mA : Sum  Inputs=+-  AccumDataTypeStr=fixdt(1, 20, 18)  OutDataTypeStr=fixdt(1, 20, 18)  SampleTime=1e-08
  p75mA : Sum  Inputs=+-  AccumDataTypeStr=fixdt(1, 19, 18)  OutDataTypeStr=fixdt(1, 19, 18)  SampleTime=1e-08
  pow2switch : Constant  OutDataTypeStr=boolean  SampleTime=1e-08
  pow2switch1 : Constant  OutDataTypeStr=boolean  SampleTime=1e-08
  x : Outport  SampleTime=1e-08
  y : Outport  Port=2  SampleTime=1e-08
  wires:
  dtc/1 -> RAMDelayBalance/1
  Amp25/1 -> QuadHandle1a/3
  Amp75/1 -> QuadHandle1b/1
  CastU16En1/1 -> CastU16En3/1
  CastU16En2/1 -> Switch/3, Saturation/1
  CastU16En3/1 -> CastU16En2/1
  GTEp75/1 -> QuadHandle1b/2, 1st or 4th Quad/2
  LTEp25/1 -> QuadHandle1a/2, 1st or 4th Quad/1
  LTEp50/1 -> QuadHandle2/2
  PipelineRegister/1 -> Positive/1, Negate/1
  Negate/1 -> SignCorrected/3
  Point25/1 -> p25mA/1, LTEp25/2, Amp25/2
  Point50/1 -> LTEp50/2
  Point75/1 -> p75mA/1, GTEp75/2, Amp75/2
  Positive/1 -> SignCorrected/1
  QuadHandle1a/1 -> QuadHandle2/1
  QuadHandle1b/1 -> QuadHandle2/3
  QuadHandle2/1 -> CastU16En1/1
  Saturation/1 -> Switch/1
  SignCorrected/1 -> y/1
  Switch/1 -> Look-Up Table/1
  insig/1 -> p75mA/2, p25mA/2, LTEp50/1, LTEp25/1, GTEp75/1, Amp75/1, Amp25/1
  p25mA/1 -> QuadHandle1a/1
  p75mA/1 -> QuadHandle1b/3
  pow2switch/1 -> Switch/2
  Amp50/1 -> QuadHandle1/3
  CastU16En21/1 -> CastU16En4/1
  CastU16En31/1 -> Switch1/3, Saturation1/1
  CastU16En4/1 -> CastU16En31/1
  LTEp251/1 -> QuadHandle21/2
  LTEp501/1 -> QuadHandle1/2, RAMDelayBalance1/1
  PipelineRegister1/1 -> Positive1/1, Negate1/1
  Negate1/1 -> SignCorrected1/3
  Point251/1 -> LTEp251/2
  Point501/1 -> p50mA/1, LTEp501/2, Amp50/2
  Positive1/1 -> SignCorrected1/1
  QuadHandle1/1 -> p50mA/2, QuadHandle21/1, LTEp251/1
  QuadHandle21/1 -> CastU16En21/1
  Saturation1/1 -> Switch1/1
  SignCorrected1/1 -> x/1
  Switch1/1 -> Look-Up Table1/1
  insig1/1 -> QuadHandle1/1, LTEp501/1, Amp50/1
  p50mA/1 -> QuadHandle21/3
  pow2switch1/1 -> Switch1/2
  1st or 4th Quad/1 -> dtc/1
  RAMDelayBalance1/1 -> SignCorrected1/2
  RAMDelayBalance/1 -> SignCorrected/2
  u/1 -> insig1/1, insig/1
  Look-Up Table/1 -> PipelineRegister/1
  Look-Up Table1/1 -> PipelineRegister1/1

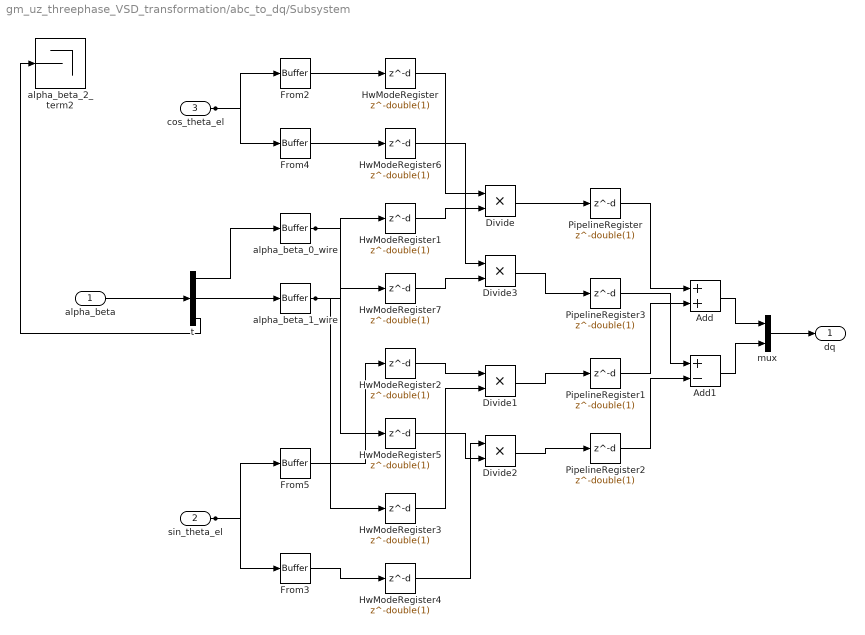
== system gm_uz_threephase_VSD_transformation/abc_to_dq/Subsystem ==
  alpha_beta : Inport  OutDataTypeStr=fixdt(1, 27, 16)  PortDimensions=[3]  SampleTime=1e-08
  sin_theta_el : Inport  Port=2  OutDataTypeStr=fixdt(1, 18, 16)  SampleTime=1e-08
  cos_theta_el : Inport  Port=3  OutDataTypeStr=fixdt(1, 18, 16)  SampleTime=1e-08
  Add : Sum  AccumDataTypeStr=fixdt(1, 28, 16)  OutDataTypeStr=fixdt(1, 27, 16)  SampleTime=1e-08
  Add1 : Sum  Inputs=+-  AccumDataTypeStr=fixdt(1, 28, 16)  OutDataTypeStr=fixdt(1, 27, 16)  SampleTime=1e-08
  Divide{,1..3} (4 alike) : Product  Inputs=**  OutDataTypeStr=fixdt(1, 27, 16)  SampleTime=1e-08
  From{2..5} (4 alike) : hdlmdlgenlib/Buffer
      settings: SourceProductBaseCode=SL
  HwModeRegister{,1..7} (8 alike) : Delay  DelayLength=double(1)  InitialCondition=0  SampleTime=1e-08
  PipelineRegister{,1..3} (4 alike) : Delay  DelayLength=double(1)  InitialCondition=0  SampleTime=1e-08
  alpha_beta_0_wire : hdlmdlgenlib/Buffer
      settings: SourceProductBaseCode=SL
  alpha_beta_1_wire : hdlmdlgenlib/Buffer
      settings: SourceProductBaseCode=SL
  alpha_beta_2_term2 : Terminator
  mux : Mux  Inputs=2
  t : Demux  Outputs=3
  dq : Outport  SampleTime=1e-08
  wires:
  Add/1 -> mux/1
  Add1/1 -> mux/2
  alpha_beta_0_wire/1 -> HwModeRegister1/1, HwModeRegister5/1
  alpha_beta_1_wire/1 -> HwModeRegister3/1, HwModeRegister7/1
  PipelineRegister/1 -> Add/1
  PipelineRegister1/1 -> Add/2
  PipelineRegister2/1 -> Add1/2
  PipelineRegister3/1 -> Add1/1
  From2/1 -> HwModeRegister/1
  From3/1 -> HwModeRegister4/1
  From4/1 -> HwModeRegister6/1
  From5/1 -> HwModeRegister2/1
  mux/1 -> dq/1
  t/1 -> alpha_beta_0_wire/1
  t/2 -> alpha_beta_1_wire/1
  t/3 -> alpha_beta_2_term2/1
  alpha_beta/1 -> t/1
  sin_theta_el/1 -> From5/1, From3/1
  cos_theta_el/1 -> From4/1, From2/1
  Divide/1 -> PipelineRegister/1
  HwModeRegister/1 -> Divide/1
  HwModeRegister1/1 -> Divide/2
  Divide1/1 -> PipelineRegister1/1
  HwModeRegister2/1 -> Divide1/1
  HwModeRegister3/1 -> Divide1/2
  Divide2/1 -> PipelineRegister2/1
  HwModeRegister4/1 -> Divide2/1
  HwModeRegister5/1 -> Divide2/2
  Divide3/1 -> PipelineRegister3/1
  HwModeRegister6/1 -> Divide3/1
  HwModeRegister7/1 -> Divide3/2

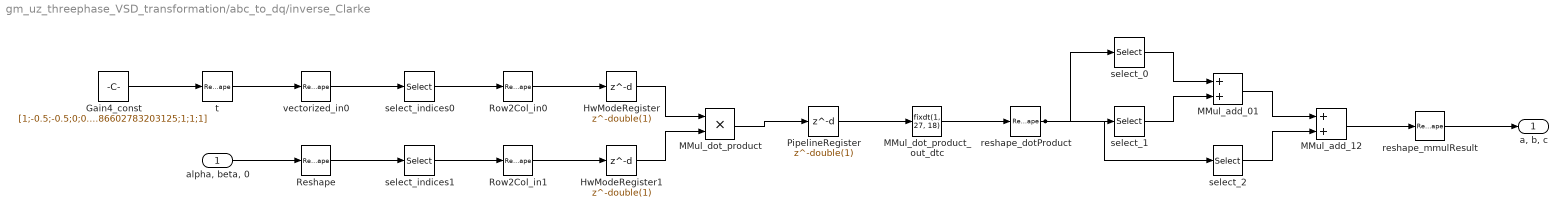
== system gm_uz_threephase_VSD_transformation/abc_to_dq/inverse_Clarke ==
  "alpha, beta, 0  " : Inport  OutDataTypeStr=fixdt(1, 27, 18)  PortDimensions=[3]  SampleTime=1e-08
  Gain4_const : Constant  Value=[1;-0.5;-0.5;0;0.86602783203125;-0.86602783203125;1;1;1]  OutDataTypeStr=fixdt(1, 18, 16)  SampleTime=1e-08
  HwModeRegister : Delay  DelayLength=double(1)  InitialCondition=0  SampleTime=1e-08
  HwModeRegister1 : Delay  DelayLength=double(1)  InitialCondition=0  SampleTime=1e-08
  MMul_add_01 : Sum  OutDataTypeStr=fixdt(1, 27, 18)  SaturateOnIntegerOverflow=on  SampleTime=1e-08
  MMul_add_12 : Sum  OutDataTypeStr=fixdt(1, 27, 18)  SaturateOnIntegerOverflow=on  SampleTime=1e-08
  MMul_dot_product : Product  Inputs=**  OutDataTypeStr=fixdt(1, 45, 34)  SampleTime=1e-08
  MMul_dot_product_out_dtc : DataTypeConversion  OutDataTypeStr=fixdt(1, 27, 18)  SampleTime=1e-08  SaturateOnIntegerOverflow=on
  PipelineRegister : Delay  DelayLength=double(1)  InitialCondition=0  SampleTime=1e-08
  Reshape : Reshape  OutputDimensionality=Column vector (2-D)
  Row2Col_in0 : Reshape  OutputDimensionality=Column vector (2-D)
  Row2Col_in1 : Reshape  OutputDimensionality=Column vector (2-D)
  reshape_dotProduct : Reshape  OutputDimensionality=Customize  OutputDimensions=[3,3]
  reshape_mmulResult : Reshape  OutputDimensionality=Customize  OutputDimensions=[3,1]
  select_0 : Selector  NumberOfDimensions=2  SampleTime=1e-08  IndexOptions=Index vector (dialog),Select all  Indices=double(1),[]  OutputSizes=1
  select_1 : Selector  NumberOfDimensions=2  SampleTime=1e-08  IndexOptions=Index vector (dialog),Select all  Indices=double(2),[]  OutputSizes=1
  select_2 : Selector  NumberOfDimensions=2  SampleTime=1e-08  IndexOptions=Index vector (dialog),Select all  Indices=double(3),[]  OutputSizes=1
  select_indices0 : Selector  SampleTime=1e-08  IndexOptions=Index vector (dialog)  Indices=double([1 4 7 2 5 8 3 6 9])  OutputSizes=1
  select_indices1 : Selector  SampleTime=1e-08  IndexOptions=Index vector (dialog)  Indices=double([1 2 3 1 2 3 1 2 3])  OutputSizes=1
  t : Reshape  OutputDimensionality=Customize  OutputDimensions=[3,3]
  vectorized_in0 : Reshape  OutputDimensionality=Row vector (2-D)
  "a, b, c" : Outport  SampleTime=1e-08
  wires:
  reshape_mmulResult/1 -> "a, b, c"/1
  Reshape/1 -> select_indices1/1
  t/1 -> vectorized_in0/1
  vectorized_in0/1 -> select_indices0/1
  select_indices0/1 -> Row2Col_in0/1
  select_indices1/1 -> Row2Col_in1/1
  Row2Col_in0/1 -> HwModeRegister/1
  Row2Col_in1/1 -> HwModeRegister1/1
  MMul_dot_product_out_dtc/1 -> reshape_dotProduct/1
  reshape_dotProduct/1 -> select_2/1, select_1/1, select_0/1
  select_0/1 -> MMul_add_01/1
  select_1/1 -> MMul_add_01/2
  MMul_add_01/1 -> MMul_add_12/1
  select_2/1 -> MMul_add_12/2
  MMul_add_12/1 -> reshape_mmulResult/1
  Gain4_const/1 -> t/1
  PipelineRegister/1 -> MMul_dot_product_out_dtc/1
  "alpha, beta, 0  "/1 -> Reshape/1
  MMul_dot_product/1 -> PipelineRegister/1
  HwModeRegister/1 -> MMul_dot_product/1
  HwModeRegister1/1 -> MMul_dot_product/2

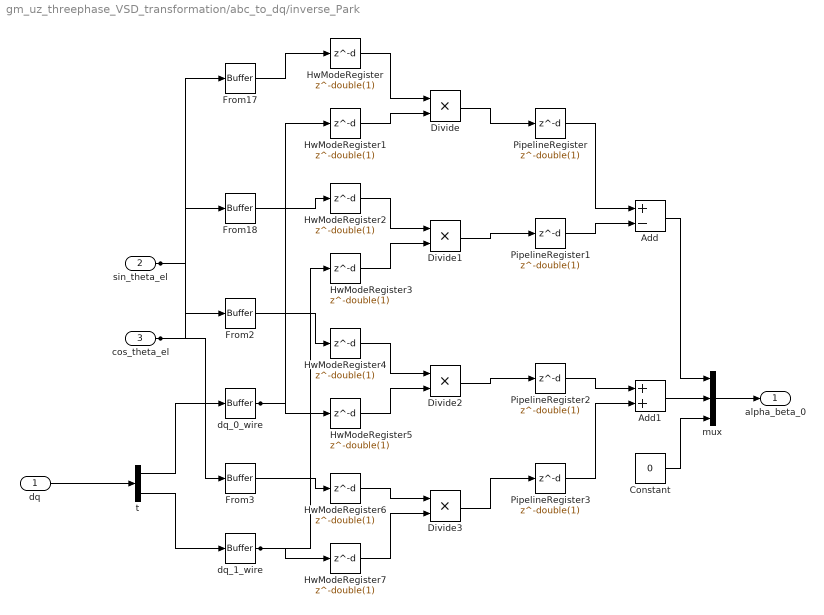
== system gm_uz_threephase_VSD_transformation/abc_to_dq/inverse_Park ==
  dq : Inport  OutDataTypeStr=fixdt(1, 27, 18)  PortDimensions=[2]  SampleTime=1e-08
  sin_theta_el : Inport  Port=2  OutDataTypeStr=fixdt(1, 18, 16)  SampleTime=1e-08
  cos_theta_el : Inport  Port=3  OutDataTypeStr=fixdt(1, 18, 16)  SampleTime=1e-08
  Add : Sum  Inputs=+-  AccumDataTypeStr=fixdt(1, 28, 18)  OutDataTypeStr=fixdt(1, 27, 18)  SampleTime=1e-08
  Add1 : Sum  AccumDataTypeStr=fixdt(1, 28, 18)  OutDataTypeStr=fixdt(1, 27, 18)  SampleTime=1e-08
  Constant : Constant  Value=0  OutDataTypeStr=fixdt(1, 27, 18)  SampleTime=1e-08
  Divide{,1..3} (4 alike) : Product  Inputs=**  OutDataTypeStr=fixdt(1, 27, 18)  SampleTime=1e-08
  From{2..3,17..18} (4 alike) : hdlmdlgenlib/Buffer
      settings: SourceProductBaseCode=SL
  HwModeRegister{,1..7} (8 alike) : Delay  DelayLength=double(1)  InitialCondition=0  SampleTime=1e-08
  PipelineRegister{,1..3} (4 alike) : Delay  DelayLength=double(1)  InitialCondition=0  SampleTime=1e-08
  dq_0_wire : hdlmdlgenlib/Buffer
      settings: SourceProductBaseCode=SL
  dq_1_wire : hdlmdlgenlib/Buffer
      settings: SourceProductBaseCode=SL
  mux : Mux  Inputs=3
  t : Demux  Outputs=2
  alpha_beta_0 : Outport  SampleTime=1e-08
  wires:
  Add/1 -> mux/1
  Add1/1 -> mux/2
  Constant/1 -> mux/3
  dq_0_wire/1 -> HwModeRegister1/1, HwModeRegister5/1
  dq_1_wire/1 -> HwModeRegister3/1, HwModeRegister7/1
  PipelineRegister/1 -> Add/1
  PipelineRegister1/1 -> Add/2
  PipelineRegister2/1 -> Add1/1
  PipelineRegister3/1 -> Add1/2
  From17/1 -> HwModeRegister/1
  From18/1 -> HwModeRegister2/1
  From2/1 -> HwModeRegister4/1
  From3/1 -> HwModeRegister6/1
  mux/1 -> alpha_beta_0/1
  t/1 -> dq_0_wire/1
  t/2 -> dq_1_wire/1
  dq/1 -> t/1
  sin_theta_el/1 -> From2/1, From18/1
  cos_theta_el/1 -> From3/1, From17/1
  Divide/1 -> PipelineRegister/1
  HwModeRegister/1 -> Divide/1
  HwModeRegister1/1 -> Divide/2
  Divide1/1 -> PipelineRegister1/1
  HwModeRegister2/1 -> Divide1/1
  HwModeRegister3/1 -> Divide1/2
  Divide2/1 -> PipelineRegister2/1
  HwModeRegister4/1 -> Divide2/1
  HwModeRegister5/1 -> Divide2/2
  Divide3/1 -> PipelineRegister3/1
  HwModeRegister6/1 -> Divide3/1
  HwModeRegister7/1 -> Divide3/2
